simulink model "PF_Balancing Simulink Model"  (R2024a)
settings: Solver=VariableStepAuto  StartTime=0.0  StopTime=inf  RelTol=1e-3
undefined symbols (not defined in the file): a, b, c
libraries: spsThreePhaseParallelRLCLoadLib x6, spsThreePhaseBreakerLib x6, spsAsynchronousMachineSIUnitsLib x1, hdlsllib x1, spsPower3phInstantaneousLib x1, spsThreePhaseVIMeasurementLib x1, sps_lib x1, spsThreePhaseSourceLib x1
settings Model: Creator=yaogu  LastModifiedBy=yaogu

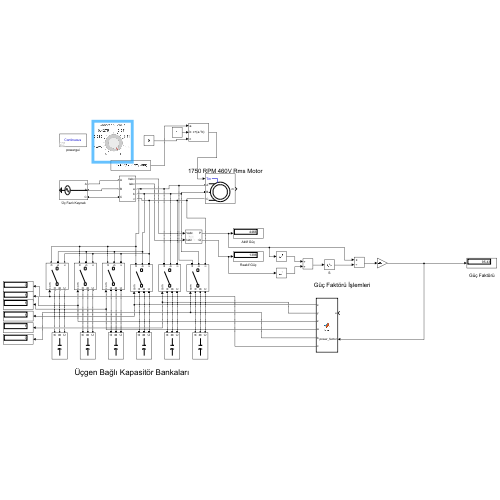
[thumbnail: Simulink's stored preview of the top-level diagram]
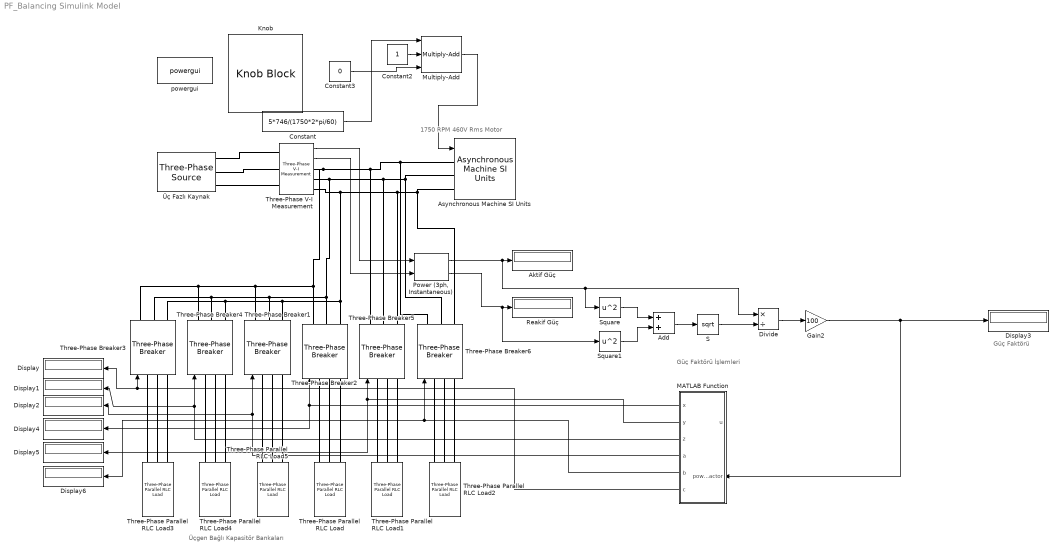
== system PF_Balancing Simulink Model ==
  note: Güç Faktörü İşlemleri
  note: Güç Faktörü
  note: Üçgen Bağlı Kapasitör Bankaları
  note: 1750 RPM 460V Rms Motor
  Add : Sum
  Aktif Güç : Display
  Asynchronous Machine SI Units : spsAsynchronousMachineSIUnitsLib/Asynchronous Machine SI Units  RotorType=Squirrel-cage  PresetModel="01:  5 HP   460 V 60Hz 1750 RPM"  MechanicalLoad=Torque Tm  ShowDetailedParameters=on  ReferenceFrame=Rotor  Units=SI  MeasurementBus=off  NominalParameters=[3730 460 60]  VoltageRatio=1  Stator=[1.115 0.005974]  Rotor=[1.083 0.005974]  Cage1=[0.4155 0.002066]  Cage2=[0.4168 0.0003495]  Lm=0.2037  Mechanical=[0.02 0.005752 2]  PolePairs=2  InitialConditions=[0 0 0 0 0 0 0 0]  SimulateSaturation=off  Saturation=[14.03593122, 27.81365428, 53.79336849, 72.68890987, 97.98006896, 148.6815601, 215.7428561, 302.9841135, 428.7778367 ; 230, 322, 414, 460, 506, 552, 598, 644, 690]  LoadFlowParameters=1492000  TsPowergui=0  TsBlock=-1  IterativeModel=Trapezoidal non iterative  IterativeDiscreteModel=Trapezoidal non iterative  Pmec=1.492e+006
  Constant : Constant  Value=5*746/(1750*2*pi/60)
  Constant2 : Constant
  Constant3 : Constant  Value=0
  Display{,1..6} (7 alike) : Display
  Divide : Product  Inputs=*/
  Gain2 : Gain  Gain=100
  Knob : KnobBlock  ScaleMax=1
  MATLAB Function : MATLAB Function  TreatAsAtomicUnit=on
  Multiply-Add : hdlsllib/HDL Operations/Multiply-Add  Function=c+(a.*b)  datatype=Inherit: Inherit via internal rule  DoSatur=off  FMA=off
  "Power (3ph, Instantaneous)" : spsPower3phInstantaneousLib/Power (3ph, Instantaneous)
  Reakif Güç : Display
  S : Sqrt
  Square : Math  Operator=square
  Square1 : Math  Operator=square
  Three-Phase Parallel RLC Load{,1,4..5} (4 alike) : spsThreePhaseParallelRLCLoadLib/Three-Phase Parallel RLC Load  LConnTagsString=A|B|C  Configuration=Delta  NominalVoltage=460  Vabc=[1e3 1e3 1e3]  Vabcp=[1e3 1e3 1e3]  NominalFrequency=60  UnbalancedPower=off  ActivePower=0  InductivePower=0  CapacitivePower=400  Pabc=[10e3 9e3 11e3]  QLabc=[100 90 110]  QCabc=[100 90 110]  Pabcp=[10e3 9e3 11e3]  QLabcp=[100 90 110]  QCabcp=[100 90 110]  Measurements=None  LoadType=constant Z
  Three-Phase Parallel RLC Load2 : spsThreePhaseParallelRLCLoadLib/Three-Phase Parallel RLC Load  LConnTagsString=A|B|C  Configuration=Delta  NominalVoltage=460  Vabc=[1e3 1e3 1e3]  Vabcp=[1e3 1e3 1e3]  NominalFrequency=60  UnbalancedPower=off  ActivePower=0  InductivePower=0  CapacitivePower=250  Pabc=[10e3 9e3 11e3]  QLabc=[100 90 110]  QCabc=[100 90 110]  Pabcp=[10e3 9e3 11e3]  QLabcp=[100 90 110]  QCabcp=[100 90 110]  Measurements=None  LoadType=constant Z
  Three-Phase Parallel RLC Load3 : spsThreePhaseParallelRLCLoadLib/Three-Phase Parallel RLC Load  LConnTagsString=A|B|C  Configuration=Delta  NominalVoltage=460  Vabc=[1e3 1e3 1e3]  Vabcp=[1e3 1e3 1e3]  NominalFrequency=60  UnbalancedPower=off  ActivePower=0  InductivePower=0  CapacitivePower=250  Pabc=[10e3 9e3 11e3]  QLabc=[100 90 110]  QCabc=[100 90 110]  Pabcp=[10e3 9e3 11e3]  QLabcp=[100 90 110]  QCabcp=[100 90 110]  Measurements=None  LoadType=constant Z
  Three-Phase V-I Measurement : spsThreePhaseVIMeasurementLib/Three-Phase V-I Measurement  VoltageMeasurement=phase-to-ground  SetLabelV=off  LabelV=Vabc  Vpu=off  VpuLL=off  CurrentMeasurement=yes  SetLabelI=off  LabelI=Iabc  Ipu=off  Pbase=100e6  Vbase=500e3  OutputType=Complex  PhasorSimulation=off  PSBequivalent=0
  Three-Phase Breaker{1..6} (6 alike) : spsThreePhaseBreakerLib/Three-Phase Breaker  InitialState=open  SwitchA=on  SwitchB=on  SwitchC=on  SwitchTimes="[1/60  5/60]"  External=on  BreakerResistance=100  SnubberResistance=inf  SnubberCapacitance=0  Measurements=None
  powergui : sps_lib/powergui  Priority=1  SimulationMode=Continuous  SampleTime=50e-6  frequency=60  Iterations=50  frequencyindice=60  Pbase=100e6  ErrMax=1e-4  UnitsV=kV  UnitsW=MW  buscounter=0  FunctionMessages=off  echomessages=off  EnableUseOfTLC=off  CurrentSourceSwitches=off  DisableSnubberDevices=off  DisableRonSwitches=off  DisableVfSwitches=off  DisplayEquations=off  AutomaticDiscreteSolvers=off  SolverType=Tustin/Backward Euler (TBE)  Interpol=off  ExternalGateDelay=off  methode=off  Ts=100  x0status=blocks  SPID=on  SwTol=0  HookPort=off  NonlinearTolerance=1e-4  nMaxIteration=100  ContinueOnMaxIteration=off  RestoreLinks=warning  ResistiveCurrentMeasurement=off  Frange=[0:2:500]  Ylog=off  Xlog=on  ShowGrid=off  save=off  variable=ZData  structure=0  ZoomFFT=off  StartTime=0.0  cycles=1  DisplayStyle=1  fundamental=60  FreqAxis=off  MaxFrequency=1000  frequencyindicesteady=1  RmsSteady=1  display=off
  Üç Fazlı Kaynak : spsThreePhaseSourceLib/Three-Phase Source  InternalConnection=Yg  VoltagePhases=off  Voltage=460  PhaseAngle=0  Voltage_phases=[25e3 25e3 25e3]/sqrt(3)  PhaseAngles_phases=[0 -120 +120]  Frequency=60  NonIdealSource=off  SpecifyImpedance=off  Resistance=0.8929  Inductance=0  ShortCircuitLevel=100e6  BaseVoltage=25e3  XRratio=7  BusType=swing  Pref=10e3  Qref=0  Prefabc=[10e3, 10e3, 10e3]  Qrefabc=[0, 0, 0]  Qmin=-inf  Qmax=inf
  wires:
  Constant/1 -> Multiply-Add/1
  Three-Phase V-I Measurement/1 -> "Power (3ph, Instantaneous)"/1
  Three-Phase V-I Measurement/2 -> "Power (3ph, Instantaneous)"/2
  "Power (3ph, Instantaneous)"/1 -> Divide/1, Square/1, Aktif Güç/1
  "Power (3ph, Instantaneous)"/2 -> Square1/1, Reakif Güç/1
  Square/1 -> Add/1
  Square1/1 -> Add/2
  Add/1 -> S/1
  S/1 -> Divide/2
  Divide/1 -> Gain2/1
  MATLAB Function/1(x) -> Three-Phase Breaker2/1, Display4/1
  MATLAB Function/2(y) -> Display5/1, Three-Phase Breaker5/1
  MATLAB Function/5(b) -> Display6/1, Three-Phase Breaker6/1
  Gain2/1 -> MATLAB Function/2(power_factor), Display3/1
  MATLAB Function/4(a) -> Display2/1, Three-Phase Breaker1/1
  MATLAB Function/6(c) -> Display/1, Three-Phase Breaker3/1
  Constant2/1 -> Multiply-Add/2
  Multiply-Add/1 -> Asynchronous Machine SI Units/1
  Constant3/1 -> Multiply-Add/3
  MATLAB Function/3(z) -> Display1/1, Three-Phase Breaker4/1
  connections:
  Üç Fazlı Kaynak/RConn1 -- Three-Phase V-I Measurement/LConn1
  Üç Fazlı Kaynak/RConn2 -- Three-Phase V-I Measurement/LConn2
  Üç Fazlı Kaynak/RConn3 -- Three-Phase V-I Measurement/LConn3
  Three-Phase V-I Measurement/RConn1 -- Three-Phase Breaker2/RConn1 -- Three-Phase Breaker1/RConn1 -- Three-Phase Breaker4/RConn1 -- Three-Phase Breaker3/RConn1 -- Three-Phase Breaker5/RConn1 -- Three-Phase Breaker6/RConn1 -- Asynchronous Machine SI Units/LConn1
  Three-Phase V-I Measurement/RConn2 -- Three-Phase Breaker2/RConn2 -- Three-Phase Breaker1/RConn2 -- Three-Phase Breaker4/RConn2 -- Three-Phase Breaker3/RConn2 -- Three-Phase Breaker5/RConn2 -- Three-Phase Breaker6/RConn2 -- Asynchronous Machine SI Units/LConn2
  Three-Phase V-I Measurement/RConn3 -- Three-Phase Breaker2/RConn3 -- Three-Phase Breaker1/RConn3 -- Three-Phase Breaker4/RConn3 -- Three-Phase Breaker3/RConn3 -- Three-Phase Breaker5/RConn3 -- Three-Phase Breaker6/RConn3 -- Asynchronous Machine SI Units/LConn3
  Three-Phase Breaker2/LConn2 -- Three-Phase Parallel RLC Load/LConn2
  Three-Phase Breaker2/LConn1 -- Three-Phase Parallel RLC Load/LConn1
  Three-Phase Breaker2/LConn3 -- Three-Phase Parallel RLC Load/LConn3
  Three-Phase Breaker5/LConn1 -- Three-Phase Parallel RLC Load1/LConn1
  Three-Phase Breaker5/LConn2 -- Three-Phase Parallel RLC Load1/LConn2
  Three-Phase Breaker5/LConn3 -- Three-Phase Parallel RLC Load1/LConn3
  Three-Phase Breaker6/LConn1 -- Three-Phase Parallel RLC Load2/LConn1
  Three-Phase Breaker6/LConn2 -- Three-Phase Parallel RLC Load2/LConn2
  Three-Phase Breaker6/LConn3 -- Three-Phase Parallel RLC Load2/LConn3
  Three-Phase Parallel RLC Load3/LConn2 -- Three-Phase Breaker3/LConn2
  Three-Phase Breaker1/LConn1 -- Three-Phase Parallel RLC Load5/LConn1
  Three-Phase Breaker1/LConn3 -- Three-Phase Parallel RLC Load5/LConn3
  Three-Phase Breaker4/LConn2 -- Three-Phase Parallel RLC Load4/LConn2
  Three-Phase Breaker1/LConn2 -- Three-Phase Parallel RLC Load5/LConn2
  Three-Phase Parallel RLC Load3/LConn1 -- Three-Phase Breaker3/LConn1
  Three-Phase Breaker3/LConn3 -- Three-Phase Parallel RLC Load3/LConn3
  Three-Phase Breaker4/LConn3 -- Three-Phase Parallel RLC Load4/LConn3
  Three-Phase Breaker4/LConn1 -- Three-Phase Parallel RLC Load4/LConn1

== matlab function PF_Balancing Simulink Model/MATLAB Function ==
  settings: updateMethod=DISCRETE  sampleTime=0.1
  data: x output; u input; y output; power_factor input; z output; a output; b output; c output
function [x, y, z, a, b, c] = fcn(u, power_factor)
    % Girişler:
    % u: Kullanılmayan giriş
    % power_factor: Mevcut güç faktörü

    % Çıkışlar:
    % x, y, z, a, b, c: Kapasitör durumları (1: Açık, 0: Kapalı)

    % Kapasitör durumlarını korumak için persistent kullanıyoruz
    persistent x_state y_state z_state a_state b_state c_state prev_power_factor;
    
    if isempty(x_state)
        % Başlangıçta tüm kapasitörler kapalı
        x_state = 0;
        y_state = 0;
        z_state = 0;
        a_state = 0;
        b_state = 0;
        c_state = 0;
        prev_power_factor = 0; % Başlangıç değeri
    end
    
    % Çıkışları mevcut durumlarla güncelle
    x = x_state;
    y = y_state;
    z = z_state;
    a = a_state;
    b = b_state;
    c = c_state;

    % Güç faktörü 93'ün üzerinde ise, kapasitörleri kapatarak 90-93 aralığına çek
    if power_factor > 98
        % Kapasitörleri sırayla kapat
        if c_state == 1
            c_state = 0; % Altıncı kapasitörü kapat
        elseif b_state == 1
            b_state = 0; % Beşinci kapasitörü kapat
        elseif a_state == 1
            a_state = 0; % Dördüncü kapasitörü kapat
        elseif z_state == 1
            z_state = 0; % Üçüncü kapasitörü kapat
        elseif y_state == 1
            y_state = 0; % İkinci kapasitörü kapat
        elseif x_state == 1
            x_state = 0; % İlk kapasitörü kapat
        end
        prev_power_factor = power_factor; % Güç faktörünü güncelle
        return;
    end

    % Güç faktörü 90'ın altında ise, kapasitörleri sıfırdan başlayarak aç
    if power_factor < 90
        % Kapasitörleri sırasıyla aç
        if x_state == 0
            x_state = 1; % İlk kapasitörü aç
        elseif y_state == 0
            y_state = 1; % İkinci kapasitörü aç
        elseif z_state == 0
            z_state = 1; % Üçüncü kapasitörü aç
        elseif a_state == 0
            a_state = 1; % Dördüncü kapasitörü aç
        elseif b_state == 0
            b_state = 1; % Beşinci kapasitörü aç
        elseif c_state == 0
            c_state = 1; % Altıncı kapasitörü aç
        end
    end

    % Güç faktörü 90 ile 93 arasında ise, kapasitör durumlarını koru
    if power_factor >= 90 && power_factor <= 93
        % Mevcut durum korunur
    end

    % Güç faktörünü güncelle
    prev_power_factor = power_factor;
end
